simulink model "testEmplanner_cs"  (R2021b)
settings: Solver=ode5  StartTime=0.0  StopTime=60  FixedStep=1/1000  RelTol=1e-3
PreLoadFcn:
  | mbxruntime.callbacks.PreLoadFcn(bdroot);
PostLoadFcn:
  | mbxruntime.callbacks.PostLoadFcn(bdroot);
InitFcn:
  | mbxruntime.callbacks.InitFcn(bdroot);
StartFcn:
  | mbxruntime.callbacks.StartFcn(bdroot);
StopFcn:
  | mbxruntime.callbacks.StopFcn(bdroot);
model workspace (MAT data in the model file):
  mbox_table : object (value not decoded)
  model_closed = 0
  sim_status = 0
values from neighbouring files (symbols this model uses):
  c_factor = 43.75    [emplanner_init.m]
  cf = -175016    [emplanner_init.m]
  cr = -130634    [emplanner_init.m]
  global_path_x = [-1.1448 -0.145417744933 0.852705365581 1.84955224935 2.84511712279 3.83939835808 4.83239585569 5.82411007764 6.81454169183 7.80369144113 8.79156009523 9.77814843293 ... (3001 elements, 3001x1)]    [global_path.mat]
  global_path_y = [14.6488 14.6488 14.6488 14.6488 14.6488 14.6488 14.6488 14.6488 14.6488 14.6488 14.6488 14.6488 ... (3001 elements, 3001x1)]    [global_path.mat]
  KD_PID_distance = 0.0    (= 0)    [emplanner_init.m]
  KD_PID_speed = 0    [emplanner_init.m]
  KI_PID_distance = 0.0    (= 0)    [emplanner_init.m]
  KI_PID_speed = 0    [emplanner_init.m]
  KP_PID_distance = 0.5    [emplanner_init.m]
  KP_PID_speed = 1.8    [emplanner_init.m]
  la = 1.265    [emplanner_init.m]
  lb = 2.947-1.265    (= 1.682)    [emplanner_init.m]
  LQR_K1 = k(:,1)'    [emplanner_init.m]
  LQR_K2 = k(:,2)'    [emplanner_init.m]
  LQR_K3 = k(:,3)'    [emplanner_init.m]
  LQR_K4 = k(:,4)'    [emplanner_init.m]
  m = 2020    [emplanner_init.m]
  rack_displacement = [-39.14 , -37.2 , -35.29 , -33.43 , -31.6 , -29.81 , -28.06 , -26.34 , -24.66 ,      -23.01 , -21.38 , -19.79 , -18.23 , -16.69 , -15.18 , -13.7 , -12.23 , -10.8 , -9.38 , -7.98 ,     -6.61 , -5.25 , -3.91 , -2.59 , -1.29 , 0 , 1.27 , 2.54 , 3.78 , 5.02 , 6.24 , 7.46 , 8.66 ,      9.86 , 11.05 , 12.24 , 13.41 , 14.59 , 15.76 , 16.92 , 18.09 , 19.25 , 20.42 , 21.59 , 22.76 ,      23.93 , 25.11 , 26 ...(+26 chars)    [emplanner_init.m]
  right_wheel_ground = [-70 ,-67.2 , -64.4 , -61.6 , -58.8 , -56 , -53.2 , -50.4 , -47.6 , -44.8 , -42 ,      -39.2 , -36.4 , -33.6 , -30.8 , -28 , -25.2 , -22.4 , -19.6 , -16.8 , -14 , -11.2 , -8.4 , -5.6 ,      -2.8 , 0 , 2.8 , 5.6 , 8.4 , 11.2 , 14 , 16.8 , 19.6 , 22.4 , 25.2 , 28 , 30.8 , 33.6 , 36.4 ,      39.2 , 42 , 44.8 , 47.6 , 50.4 , 53.2 , 56 , 58.8 , 61.6 , 64.4 , 67.2 , 70 ]    [emplanner_init.m]
  vx_break_point = zeros(1,5000)    [emplanner_init.m]
undefined symbols (not defined in the file or in its folder): aubr, DiscIntNeverNeededParam, tablebr, vubr, warningInitialVelocity, x0
libraries: simulink x19, PreScanSimulinkLibrary x17, simulink_extras x6, Solver_SF x1
(part 10 of 14)

== matlab function testEmplanner_cs/Audi_A8_Sedan_1/decision&planning module/EM Planner/decesion task/path decision with dynamic planning(dp) ==
  data: obs_s_set input; dp_path_s output; obs_l_set input; plan_start_s input; plan_start_l input; plan_start_dl input; plan_start_dll input; w_cost_collision input; w_cost_smooth_dl input; w_cost_smooth_ddl input; w_cost_smooth_dddl input; w_cost_ref input; row input; col input; sample_s input; sample_l input; dp_path_l output
function [dp_path_s,dp_path_l] = fcn(obs_s_set,obs_l_set,plan_start_s,plan_start_l,plan_start_dl,...
    plan_start_dll,w_cost_collision,w_cost_smooth_dl,w_cost_smooth_ddl,w_cost_smooth_dddl,w_cost_ref,row,col,sample_s,sample_l)
%该函数为路径决策算法动态规划的主函数
% 输入：obs s l set 筛选后的障碍物sl信息
%       plan_start s l dl ddl 规划起点信息
%       w_cost_obs,w_cost_smooth_dl,w_cost_smooth_ddl,w_cost_smooth_dddl,w_cost_ref动态规划代价权重
%       row col 动态规划采样点的行数和列数(row必须是奇数，col必须是6)
%       sample_s,sample_l 采样的s l 长度
% 输出：dp_path_l,dp_path_s 动态规划的路径sl,此路径不包含规划起点  

%动态规划最优的数据结构是结构体矩阵，但是simulink不支持结构体矩阵，所以动态规划算法写的相对难以理解

%声明二维矩阵变量node_cost，node_cost(i,j)表示从起点出发，到行i列j节点的最小代价为node_cost(i,j)
node_cost = ones(row,col)*inf;%初始化为无穷大

%声明二维矩阵变量pre_node_index pre_node_index(i,j)表示从起点到行i列j的节点的最优路径中前一个节点的行号为
%pre_node_index(i,j)
%例：比如一条最优路径为 起点 -> node(1,1) -> node(2,2) -> node(3,3)
%则pre_node_index(3,3) = 2 (最优路径的前一个节点是node(2,2) 取它的行号）
%  pre_node_index(2,2) = 1 (最优路径的前一个节点是node(1,1) 取它的行号）
%  pre_node_index(1,1) = 0 (起点的行号默认是0)

% 其实pre_node_index就是当找到最小代价的路径后从终点到起点反向选择出最优路径的
%如果用结构体矩阵完全没有必要弄得这么麻烦，但是simulink不支持
pre_node_index = zeros(row,col);%初始化，所有节点的上个最优节点的行号都是0，也就是起点

%先计算从起点到第一列的cost
for i = 1:row
    node_cost(i,1) = CalcStartCost(plan_start_s,plan_start_l,plan_start_dl,...
    plan_start_dll,i,sample_s,sample_l,w_cost_collision,w_cost_smooth_dl,...
    w_cost_smooth_ddl,w_cost_smooth_dddl,w_cost_ref,obs_s_set,obs_l_set,row);
end
% 动态规划主函数，从第二列开始
for j = 2:col
    for i = 1:row
        %计算当前node(i,j)的s l
        cur_node_s = plan_start_s + j * sample_s;
        cur_node_l = ((row + 1)/2 - i) * sample_l;
        %遍历前一列的节点
        for k = 1:row
            %计算前一列节点的s l
            pre_node_s = plan_start_s + (j - 1) * sample_s;
            pre_node_l = ((row + 1)/2 - k) * sample_l;
            cost_neighbour = CalcNeighbourCost(pre_node_s,pre_node_l,cur_node_s,cur_node_l,w_cost_collision,...
    w_cost_smooth_dl,w_cost_smooth_ddl,w_cost_smooth_dddl,w_cost_ref,obs_s_set,obs_l_set);
            %起点到上一个节点的最小代价为node_cost(k,j-1)
            pre_min_cost = node_cost(k,j-1);
            %起点到node_cost(i,j)的最小代价 为node_cost(k,j-1)
            %再加上node(k,j-1)到node(i,j)的代价 (k = 1,2,3,4...row) 中最小的
            cost_temp = pre_min_cost + cost_neighbour;
            if cost_temp < node_cost(i,j)
                node_cost(i,j) = cost_temp;
                %把最优路径上一列节点的行号记录下来
                pre_node_index(i,j) = k;
            end
        end      
    end
end
%找到node_cost最后一列中，cost最小的，记代价最小的行号为index
index = 0;
min_cost = inf;
for i = 1:row
    if node_cost(i,end) < min_cost
        min_cost = node_cost(i,end);
        index = i;
    end
end
%动态规划最优路径初始化
dp_node_list_row = zeros(col,1);
%从后往前逆推
cur_index = index;
for i = 1:col
    %记录cur_index前面节点的行号
    pre_index = pre_node_index(cur_index,end - i + 1);
    %把cur_index放到dp_node_list_row对应的位置
    dp_node_list_row(col - i + 1) = cur_index;
    %再把pre_index 赋给 cur_index 进行下一步递推
    cur_index = pre_index;
end
% 输出初始化，由于事先不知道横纵向的采样列数，因此需要做缓冲
dp_path_s = ones(15,1)*-1;
dp_path_l = ones(15,1)*-1;
for i = 1:col
    dp_path_s(i) = plan_start_s + i * sample_s;
    dp_path_l(i) = ((row + 1) / 2 - dp_node_list_row(i)) * sample_l;
end








end
function cost = CalcNeighbourCost(pre_node_s,pre_node_l,cur_node_s,cur_node_l,w_cost_collision,...
    w_cost_smooth_dl,w_cost_smooth_ddl,w_cost_smooth_dddl,w_cost_ref,obs_s_set,obs_l_set)
% 该函数将计算相邻两个节点之间的cost
  
    start_l = pre_node_l;
    start_dl = 0;
    start_ddl = 0;
    end_l = cur_node_l;
    end_dl = 0;
    end_ddl = 0;
    start_s = pre_node_s;
    end_s = cur_node_s;
    coeff = CalcQuinticCoeffient(start_l,start_dl,start_ddl,end_l,end_dl,end_ddl,start_s,end_s);
    a0 = coeff(1);
    a1 = coeff(2);
    a2 = coeff(3);
    a3 = coeff(4);
    a4 = coeff(5);
    a5 = coeff(6);
    % 取10个点计算cost
    ds = zeros(10,1);
    l = zeros(10,1);
    dl = zeros(10,1);
    ddl = zeros(10,1);
    dddl = zeros(10,1);
    for i = 1:10
        ds(i) = start_s + (i-1)*(end_s - start_s)/10;
    end
    l = a0 * ones(10,1) + a1 * ds + a2 * ds.^2 + a3 * ds.^3 + a4 * ds.^4 + a5 * ds.^5;
    dl = a1 * ones(10,1) + 2 * a2 * ds + 3 * a3 * ds.^2 + 4 * a4 * ds.^3 + 5 * a5 * ds.^4;
    ddl = 2 * a2 * ones(10,1) + 6 * a3 * ds + 12 * a4 * ds.^2 + 20 * a5 * ds.^3;
    dddl = 6 * ones(10,1) * a3 + 24 * a4 * ds + 60 * a5 * ds.^2;
    cost_smooth = w_cost_smooth_dl * (dl' * dl) + w_cost_smooth_ddl * (ddl' * ddl) + w_cost_smooth_dddl * (dddl' * dddl);
    cost_ref = w_cost_ref * (l' * l);
    cost_collision = 0;
    for i = 1:length(obs_s_set)
        if isnan(obs_s_set(i))
            break;
        end
        dlon = ones(10,1) * obs_s_set(i) - ds;
        dlat = ones(10,1) * obs_l_set(i) - l;
        %这里做了非常简化的质点模型，认为障碍物就是一个点
        square_d = dlon.^2 + dlat.^2;
        cost_collision_once = CalcObsCost(w_cost_collision,square_d);
        cost_collision = cost_collision + cost_collision_once;
    end
    cost = cost_collision + cost_smooth + cost_ref;


end


function cost = CalcStartCost(begin_s,begin_l,begin_dl,begin_ddl,cur_node_row,sample_s,sample_l,w_cost_collision,...
    w_cost_smooth_dl,w_cost_smooth_ddl,w_cost_smooth_dddl,w_cost_ref,obs_s_set,obs_l_set,row)
    %该函数将计算起点到第一层的cost
    start_l = begin_l;
    start_dl = begin_dl;
    start_ddl = begin_ddl;
    %  . . .
    %  . . . row = 3 中间的行号 = (row + 1) /2 = 2
    %  . . .
    end_l = ((row + 1)/2 - cur_node_row)*sample_l;
    end_dl = 0;
    end_ddl = 0;
    start_s = begin_s;
    end_s = begin_s + sample_s;
    coeff = CalcQuinticCoeffient(start_l,start_dl,start_ddl,end_l,end_dl,end_ddl,start_s,end_s);
    a0 = coeff(1);
    a1 = coeff(2);
    a2 = coeff(3);
    a3 = coeff(4);
    a4 = coeff(5);
    a5 = coeff(6);
    % 取10个点计算cost
    ds = zeros(10,1);
    l = zeros(10,1);
    dl = zeros(10,1);
    ddl = zeros(10,1);
    dddl = zeros(10,1);
    for i = 1:10
        ds(i) = start_s + (i-1)*sample_s/10;
    end
    l = a0 * ones(10,1) + a1 * ds + a2 * ds.^2 + a3 * ds.^3 + a4 * ds.^4 + a5 * ds.^5;
    dl = a1 * ones(10,1) + 2 * a2 * ds + 3 * a3 * ds.^2 + 4 * a4 * ds.^3 + 5 * a5 * ds.^4;
    ddl = 2 * a2 * ones(10,1) + 6 * a3 * ds + 12 * a4 * ds.^2 + 20 * a5 * ds.^3;
    dddl = 6 * ones(10,1) * a3 + 24 * a4 * ds + 60 * a5 * ds.^2;
    cost_smooth = w_cost_smooth_dl * (dl' * dl) + w_cost_smooth_ddl * (ddl' * ddl) + w_cost_smooth_dddl * (dddl' * dddl);
    cost_ref = w_cost_ref * (l' * l);
    cost_collision = 0;
    for i = 1:length(obs_s_set)
        if isnan(obs_s_set(i))
            break;
        end
        dlon = ones(10,1) * obs_s_set(i) - ds;
        dlat = ones(10,1) * obs_l_set(i) - l;
        %这里做了非常简化的质点模型，认为障碍物就是一个点
        square_d = dlon.^2 + dlat.^2;
        cost_collision_once = CalcObsCost(w_cost_collision,square_d);
        cost_collision = cost_collision + cost_collision_once;
    end
    cost = cost_collision + cost_smooth + cost_ref;
        
end

function obs_cost = CalcObsCost(w_cost_collision,square_d)
%该函数将计算障碍物的距离代价
% 暂定超过4米的cost为0 在4到3米的cost为1000/squard_d,在小于3米的cost为w_cost_collision
  cost = 0;
  for i = 1:length(square_d)
      if (square_d(i) < 16 && square_d(i) > 9) 
          cost = cost + 1000/square_d(i);
      elseif (square_d(i) < 9)
          cost = cost + w_cost_collision;
      end
  end
  obs_cost = cost;

end

function coeff = CalcQuinticCoeffient(start_l,start_dl,start_ddl,end_l,end_dl,end_ddl,start_s,end_s)
    % l = a0 + a1*s + a2*s^2 + a3*s^3 + a4*s^4 + a5*s^5
    % l' = a1 + 2 * a2 * s + 3 * a3 * s^2 + 4 * a4 * s^3 + 5 * a5 * s^4
    % l'' = 2 * a2 + 6 * a3 * s + 12 * a4 * s^2 + 20 * a5 * s^3
    start_s2 = start_s * start_s;
    start_s3 = start_s2 * start_s;
    start_s4 = start_s3 * start_s;
    start_s5 = start_s4 * start_s;
    end_s2 = end_s * end_s;
    end_s3 = end_s2 * end_s;
    end_s4 = end_s3 * end_s;
    end_s5 = end_s4 * end_s;
    A = [1,start_s, start_s2,     start_s3,     start_s4,      start_s5;
         0 1,       2 * start_s,  3 * start_s2, 4 * start_s3,  5 * start_s4;
         0 0,       2,            6 * start_s,  12 * start_s2, 20 * start_s3;
         1,end_s, end_s2,     end_s3,     end_s4,      end_s5;
         0,1,     2 * end_s,  3 * end_s2, 4 * end_s3,  5 * end_s4;
         0,0,     2,          6 * end_s,  12 * end_s2, 20 * end_s3;];
    B = [start_l;
         start_dl;
         start_ddl;
         end_l;
         end_dl;
         end_ddl;];
     coeff = A \ B;
    
end

== matlab function testEmplanner_cs/Audi_A8_Sedan_1/decision&planning module/referenceline provider/MATLAB Function ==
  data: x_set input; match_point_index_set output; y_set input; frenet_path_x input; frenet_path_y input; frenet_path_heading input; frenet_path_kappa input; proj_x_set output; proj_y_set output; proj_heading_set output; proj_kappa_set output
function [match_point_index_set,proj_x_set,proj_y_set,proj_heading_set,proj_kappa_set] = ...
	fcn(x_set,y_set,frenet_path_x,frenet_path_y,frenet_path_heading,frenet_path_kappa)
	
%该函数将批量计算x_set,y_set中(x,y) 在frenet坐标系下的投影信息
%输入： x_set，y_set 待投影的点的集合
	%x_set,y_set,frenet_path_x,frenet_path_y,frenet_path_heading,frenet_path_kappa
	%曲线在直角坐标系下的x,y,heading,kappa
%输出：math_point_index_set 匹配点在frenet_path下的编号的集合（即从全局路径的第一个点开始数，第几个点是匹配点）

%由于事先不知道x_set中有多少个点需要投影，因此事先声明一个最大数量的点作为缓冲

n = 128;
%并且不知道投影点的数量，所以也不知道输出的数量，因此输出也要做缓冲，用nan表示不存在的点
%初始化输出最多为128个点。
%输出初始化
match_point_index_set = ones(n,1) * nan;
proj_x_set = ones(n,1) * nan;
proj_y_set = ones(n,1) * nan;
proj_heading_set = ones(n,1) * nan;
proj_kappa_set = ones(n,1) * nan;

%找匹配点，需要利用上一个周期的结果作为下一个周期遍历的起点，因此需要声明两个全局变量
persistent is_first_run;
persistent pre_match_point_index_set;%bug :pre_match_point_index(i) 未必代表的是第i个障碍物的match_point_index
persistent pre_frenet_path_x;
persistent pre_frenet_path_y;
persistent pre_frenet_path_heading;
persistent pre_frenet_path_kappa;
persistent pre_x_set;
persistent pre_y_set;
%算法主函数入口

if isempty(is_first_run)
	% 该if分支表示函数首次运行
	is_first_run = 0; %赋值
	pre_frenet_path_x = frenet_path_x;
	pre_frenet_path_y = frenet_path_y;
	pre_frenet_path_heading = frenet_path_heading;
	pre_frenet_path_kappa = frenet_path_kappa;
	%记录首次运行计算的匹配点的结果供下个周期运行，先初始化
	pre_match_point_index_set = ones(n,1) * nan;
	
	%对x_set,y_set的点做遍历，找到他们的匹配点
	for i = 1 : length(x_set)
        if isnan(x_set(i))
            break;
        end
	%首次运行时，没有任何提示，只能从frenet_path的第一个点开始找
	start_search_index = 1;
	%声明increa_count,用于表示在遍历时distance连续增大的次数
	increase_count = 0;
	%开始遍历
	min_distance = inf;
	for j = start_search_index : length(frenet_path_x)
		distance = (x_set(i) - frenet_path_x(j))^2 + (y_set(i) - frenet_path_y(j))^2;
		%处理最小值
		if distance < min_distance
			min_distance = distance;
			match_point_index_set(i) = j; %math_point_index_set存放匹配点的序号
			increase_count = 0;
		else
			increase_count = increase_count + 1;
		end
		% 如果连续distanc增加50次,就不要再遍历了，节省时间
		if increase_count > 50 
			break;
		end	
	end
	%如何通过匹配点计算投影点，参考《自动驾驾驶控制算法第七讲》
	%或者《自动驾驶决策规划算法》第一章第三节
		
	%取出匹配点的编号
	match_point_index = match_point_index_set(i);
		
	%取出匹配点信息
	match_point_x = frenet_path_x(match_point_index);
	match_point_y = frenet_path_y(match_point_index);
	match_point_heading = frenet_path_heading(match_point_index);
	match_point_kappa = frenet_path_kappa(match_point_index);
		
	% 计算匹配点的位置向量和方向向量
	vector_match_point = [match_point_x;match_point_y];%位置向量
	vector_match_point_direction = [cos(match_point_heading);sin(match_point_heading)];%方向向量，全局坐标系下（大地坐标系）
		
	%声明待投影点的位矢
	vector_r = [x_set(i);y_set(i)];
		
	%通过匹配点计算投影点
	vector_d = vector_r - vector_match_point;
	ds = vector_d' * vector_match_point_direction;
	vector_proj_point = vector_match_point + ds * vector_match_point_direction;
	proj_heading = match_point_heading + match_point_kappa * ds;
	proj_kappa = match_point_kappa;
		
	%计算结果输出 
	proj_x_set(i) = vector_proj_point(1);
	proj_y_set(i) = vector_proj_point(2);
	proj_heading_set(i) = proj_heading;
	proj_kappa_set(i) = proj_kappa;
   end
	
	%匹配点的计算结果保存，供下一个周期使用
	pre_match_point_index_set = match_point_index_set;
	pre_x_set = x_set;
	pre_y_set = y_set;
else
	% 此分支不是首次运行
	
	%对每个x_set上的点做处理
	for i = 1 : length(x_set)
		%不是首次运行，对于点x_set(i),y_set(i)来说，
		%start_search_index = pre_match_point_index_set(i)
		start_search_index = pre_match_point_index_set(i);%上个周期匹配点的编号作为本周期搜索的起点
		%判断帧与帧之间的障碍物是否为同一个
		square_dis = (x_set(i) - pre_x_set(i))^2 + (y_set(i) - pre_y_set(i))^2;
		if square_dis > 36	 
			% 帧与帧之间的物体位置距离过大，认为是两个障碍物
			start_search_index = nan;
		end
        %
        % 对于障碍物的检测而言，当感知第一次检测到障碍物时，算法并不是首次运行，此时
        % pre_match_point_set的值是nan，如果还用上一个时刻的结果作为本周期搜索的起点
        % 必然会出问题，所以要修改
        % 声明 increase_count_limit
        increase_count_limit = 5;
        if isnan(start_search_index)
	        % 没有上个周期的结果，那么就不能只检查5次
	        increase_count_limit = 50;
	        % 搜索的起点也要设为 1
	        start_search_index = 1;
        end
		%声明increa_count,用于表示在遍历时distance连续增大的次数
		increase_count = 0;
		%开始遍历
		
		%这里多了一个步骤，判断遍历的方向
		%计算上个周期匹配点的位失
		vector_pre_match_point = [pre_frenet_path_x(start_search_index); pre_frenet_path_y(start_search_index)];
		vector_pre_match_point_direction = ...
			[cos(pre_frenet_path_heading(start_search_index));sin(pre_frenet_path_heading(start_search_index))];
		
		% 判断遍历的方向
		flag = ([x_set(i);y_set(i)] - vector_pre_match_point)' * vector_pre_match_point_direction;
		
		min_distance = inf;
		
		if flag > 0.001 
			for j = start_search_index : length(frenet_path_x)
				distance = (x_set(i) - frenet_path_x(j))^2 + (y_set(i) - frenet_path_y(j))^2;
				%处理最小值
				if distance < min_distance
					min_distance = distance;
					match_point_index_set(i) = j; %math_point_index_set存放匹配点的序号
					increase_count = 0;
				else
					increase_count = increase_count + 1;
				end
				% 如果连续distanc增加increase_count_limit次,就不要再遍历了，节省时间
				if increase_count > increase_count_limit
					break;
				end
			end
		elseif flag < -0.001
			for j = start_search_index :-1: 1
				distance = (x_set(i) - frenet_path_x(j))^2 + (y_set(i) - frenet_path_y(j))^2;
				%处理最小值
				if distance < min_distance
					min_distance = distance;
					match_point_index_set(i) = j; %math_point_index_set存放匹配点的序号
					increase_count = 0;
				else
					increase_count = increase_count + 1;
				end
				% 如果连续distanc增加50次,就不要再遍历了，节省时间
				if increase_count > increase_count_limit 
					break;
				end
			end
		else
			match_point_index_set(i) = start_search_index;
		end
			
		%如何通过匹配点计算投影点，参考《自动驾驾驶控制算法第七讲》
		%或者《自动驾驶决策规划算法》第一章第三节
		
		%取出匹配点的编号
		match_point_index = match_point_index_set(i);
		
		%取出匹配点信息
		match_point_x = frenet_path_x(match_point_index);
		match_point_y = frenet_path_y(match_point_index);
		match_point_heading = frenet_path_heading(match_point_index);
		match_point_kappa = frenet_path_kappa(match_point_index);
		
		% 计算匹配点的位置向量和方向向量
		vector_match_point = [match_point_x;match_point_y];%位置向量
		vector_match_point_direction = [cos(match_point_heading);sin(match_point_heading)];%方向向量
		
		%声明待投影点的位矢
		vector_r = [x_set(i);y_set(i)];
		
		%通过匹配点计算投影点
		vector_d = vector_r - vector_match_point;
		ds = vector_d' * vector_match_point_direction;
		vector_proj_point = vector_match_point + ds * vector_match_point_direction;
		proj_heading = match_point_heading + match_point_kappa * ds;
		proj_kappa = match_point_kappa;
		
		%计算结果输出 
		proj_x_set(i) = vector_proj_point(1);
		proj_y_set(i) = vector_proj_point(2);
		proj_heading_set(i) = proj_heading;
		proj_kappa_set(i) = proj_kappa;
	end
	
	%匹配点的计算结果保存，供下一个周期使用
	pre_match_point_index_set = match_point_index_set;
	pre_frenet_path_x = frenet_path_x;
	pre_frenet_path_y = frenet_path_y;
	pre_frenet_path_heading = frenet_path_heading;
	pre_frenet_path_kappa = frenet_path_kappa;
	pre_x_set = x_set;
	pre_y_set = y_set;
end

== matlab function testEmplanner_cs/Audi_A8_Sedan_1/decision&planning module/EM Planner/decesion task/increase DP path nodes ==
  data: dp_path_s_init input; dp_path_s_final output; dp_path_l_init input; plan_start_s input; plan_start_l input; plan_start_dl input; plan_start_ddl input; dp_path_l_final output; dp_path_dl_final output; dp_path_ddl_final output
function [dp_path_s_final,dp_path_l_final,dp_path_dl_final,dp_path_ddl_final] = ... 
	fcn(dp_path_s_init,dp_path_l_init,plan_start_s,plan_start_l,plan_start_dl,plan_start_ddl)
% 该函数将增密dp_path_s,dp_path_l
% 由于事先不知道动态规划采样的行和列，也就不知道动态规划计算的曲线有多长，因此需要做缓冲
% 每1“米” 采样一个点，一共60个
ds = 1;
% 输出初始化
dp_path_s_final = ones(60,1) * nan;
dp_path_l_final = ones(60,1) * nan;
dp_path_dl_final = ones(60,1) * nan;
dp_path_ddl_final = ones(60,1) * nan;

% 设置五次多项式的起点
start_s = plan_start_s;
start_l = plan_start_l;
start_dl = plan_start_dl;
start_ddl = plan_start_ddl;

s_cur = [];
l_temp = [];
dl_temp = [];
ddl_temp = [];

for i = 1 : length(dp_path_s_init)
	if isnan(dp_path_s_init(i)) 
		break;
	end
	for j = 1 : 1000
		% 采样s
		s_node = start_s + ds * (j - 1);
		if s_node < dp_path_s_init(i)
			s_cur = [s_cur,s_node];% 矩阵动态扩容
		else
			break;
		end

	end
	end_s = dp_path_s_init(i);
	end_l = dp_path_l_init(i);
	end_dl = 0;
	end_ddl = 0;
	coeff = CalcQuinticCoeffient(start_l,start_dl,start_ddl,end_l,end_dl,end_ddl,start_s,end_s);
	a0 = coeff(1);
	a1 = coeff(2);
	a2 = coeff(3);
	a3 = coeff(4);
	a4 = coeff(5);
	a5 = coeff(6);
	l = a0 * ones(1,length(s_cur)) + a1 * s_cur + a2 * s_cur.^2 + a3 * s_cur.^3 +...
		a4 * s_cur.^4 + a5 * s_cur.^5 ;
	dl = a1 * ones(1,length(s_cur)) + 2 * a2 * s_cur + 3 * a3 * s_cur.^2 + ...
		4 * a4 * s_cur.^3 + 5 * a5 * s_cur.^4;
	ddl = 2 * a2 * ones(1,length(s_cur)) + 6 * a3 * s_cur + ...
		12 * a4 * s_cur.^2 + 20 * a5 * s_cur.^3;
	% 把 l dl ddl 的结果保存
	l_temp = [l_temp,l];
	dl_temp = [dl_temp,dl];
	ddl_temp = [ddl_temp,ddl];
	% end的值 赋值给start做下一步循环使用
	start_s = end_s;
	start_l = end_l;
	start_dl = end_dl;
	start_ddl = end_ddl;
	s_cur = [];% 清空临时数组
end

	for k = 1 : length(l_temp)
		if k == 61 
			break;
		end

		dp_path_s_final(k) = plan_start_s + ds * (k - 1);
		dp_path_l_final(k) = l_temp(k);
		dp_path_dl_final(k) = dl_temp(k);
		dp_path_ddl_final(k) = ddl_temp(k);

	end

end


function coeff = CalcQuinticCoeffient(start_l,start_dl,start_ddl,end_l,end_dl,end_ddl,start_s,end_s)
	% l = a0 + a1 * s + a2 * s^2 + a3 * s^3 + a4 * s^4 + a5 * s^5;
	% l' = a1 + 2 * a2 * s + 3 * a3 * s^2 + 4 * a4 * s^3 + 5 * a5 * s^4;
	% l'' = 2 * a2 + 6 * a3 * s + 12 * a4 * s^2 + 20 * a5 * s^3;
	start_s2 = start_s * start_s;
	start_s3 = start_s2 * start_s;
	start_s4 = start_s3 * start_s;
	start_s5 = start_s4 * start_s;

	end_s2 = end_s * end_s;
	end_s3 = end_s2 * end_s;
	end_s4 = end_s3 * end_s;
	end_s5 = end_s4 * end_s;
	% 构造A B矩阵，然后求方程的系数即可

	A = [ 1, start_s, start_s2,  start_s3,   start_s4,   start_s5;
		  0 , 1     , 2*start_s, 3*start_s2, 4*start_s3,  5*start_s4;
		  0 , 0     , 2        , 6*start_s,  12*start_s2, 20*start_s3;
		  1, end_s, end_s2,  end_s3,   end_s4,   end_s5;
		  0 , 1     , 2*end_s, 3*end_s2, 4*end_s3,  5*end_s4;
		  0 , 0     , 2       , 6*end_s,  12*end_s2, 20*end_s3;
		];
	B = [ start_l;
		  start_dl;
		  start_ddl;
		  end_l;
		  end_dl;
		  end_ddl;
		];
	coeff = A \ B;
end

== matlab function testEmplanner_cs/Audi_A8_Sedan_1/decision&planning module/EM Planner/MATLAB Function3 ==
  data: dp_speed_s input; dp_speed_t input; qp_speed_s input; qp_speed_t input; obs_s_in_set input; obs_s_out_set input; obs_t_in_set input; obs_t_out_set input
function  fcn(dp_speed_s,dp_speed_t,qp_speed_s,qp_speed_t,obs_s_in_set,obs_s_out_set,obs_t_in_set,obs_t_out_set)
coder.extrinsic("plot");
cla;
n = length(dp_speed_s);
m = length(obs_s_in_set);
s = length(qp_speed_s);
for i = 1:length(dp_speed_s)
    if isnan(dp_speed_s(i))
        n = i -1;
        break;
    end
end
for i = 1:length(qp_speed_s)
    if isnan(qp_speed_s(i))
        s = i -1;
        break;
    end
end

plot(dp_speed_t(1:n),dp_speed_s(1:n),'r')
plot(qp_speed_t(1:s),qp_speed_s(1:s),'b')
hold on
axis([-1 10 -10 50]);
for i = 1:m
    if isnan(obs_s_in_set(i))
        continue;
    end
    point_t = [obs_t_in_set(i),obs_t_out_set(i)];
    point_s = [obs_s_in_set(i),obs_s_out_set(i)];
    plot(point_t,point_s)
end

== matlab function testEmplanner_cs/Audi_A8_Sedan_1/decision&planning module/EM Planner/MATLAB Function5 ==
  data: x_set input; match_point_index_set output; y_set input; frenet_path_x input; frenet_path_y input; frenet_path_heading input; frenet_path_kappa input; proj_x_set output; proj_y_set output; proj_heading_set output; proj_kappa_set output
function [match_point_index_set,proj_x_set,proj_y_set,proj_heading_set,proj_kappa_set] = ...
	fcn(x_set,y_set,frenet_path_x,frenet_path_y,frenet_path_heading,frenet_path_kappa)
	
%该函数将批量计算x_set,y_set中(x,y) 在frenet坐标系下的投影信息
%输入： x_set，y_set 待投影的点的集合
	%x_set,y_set,frenet_path_x,frenet_path_y,frenet_path_heading,frenet_path_kappa
	%曲线在直角坐标系下的x,y,heading,kappa
%输出：math_point_index_set 匹配点在frenet_path下的编号的集合（即从全局路径的第一个点开始数，第几个点是匹配点）

%由于事先不知道x_set中有多少个点需要投影，因此事先声明一个最大数量的点作为缓冲

n = 128;
%并且不知道投影点的数量，所以也不知道输出的数量，因此输出也要做缓冲，用nan表示不存在的点
%初始化输出最多为128个点。
%输出初始化
match_point_index_set = ones(n,1) * nan;
proj_x_set = ones(n,1) * nan;
proj_y_set = ones(n,1) * nan;
proj_heading_set = ones(n,1) * nan;
proj_kappa_set = ones(n,1) * nan;

%找匹配点，需要利用上一个周期的结果作为下一个周期遍历的起点，因此需要声明两个全局变量
persistent is_first_run;
persistent pre_match_point_index_set;%bug :pre_match_point_index(i) 未必代表的是第i个障碍物的match_point_index
persistent pre_frenet_path_x;
persistent pre_frenet_path_y;
persistent pre_frenet_path_heading;
persistent pre_frenet_path_kappa;
persistent pre_x_set;
persistent pre_y_set;
%算法主函数入口

if isempty(is_first_run)
	% 该if分支表示函数首次运行
	is_first_run = 0; %赋值
	pre_frenet_path_x = frenet_path_x;
	pre_frenet_path_y = frenet_path_y;
	pre_frenet_path_heading = frenet_path_heading;
	pre_frenet_path_kappa = frenet_path_kappa;
	%记录首次运行计算的匹配点的结果供下个周期运行，先初始化
	pre_match_point_index_set = ones(n,1) * nan;
	
	%对x_set,y_set的点做遍历，找到他们的匹配点
	for i = 1 : length(x_set)
        if isnan(x_set(i))
            break;
        end
	%首次运行时，没有任何提示，只能从frenet_path的第一个点开始找
	start_search_index = 1;
	%声明increa_count,用于表示在遍历时distance连续增大的次数
	increase_count = 0;
	%开始遍历
	min_distance = inf;
	for j = start_search_index : length(frenet_path_x)
		distance = (x_set(i) - frenet_path_x(j))^2 + (y_set(i) - frenet_path_y(j))^2;
		%处理最小值
		if distance < min_distance
			min_distance = distance;
			match_point_index_set(i) = j; %math_point_index_set存放匹配点的序号
			increase_count = 0;
		else
			increase_count = increase_count + 1;
		end
		% 如果连续distanc增加50次,就不要再遍历了，节省时间
		if increase_count > 50 
			break;
		end	
	end
	%如何通过匹配点计算投影点，参考《自动驾驾驶控制算法第七讲》
	%或者《自动驾驶决策规划算法》第一章第三节
		
	%取出匹配点的编号
	match_point_index = match_point_index_set(i);
		
	%取出匹配点信息
	match_point_x = frenet_path_x(match_point_index);
	match_point_y = frenet_path_y(match_point_index);
	match_point_heading = frenet_path_heading(match_point_index);
	match_point_kappa = frenet_path_kappa(match_point_index);
		
	% 计算匹配点的位置向量和方向向量
	vector_match_point = [match_point_x;match_point_y];%位置向量
	vector_match_point_direction = [cos(match_point_heading);sin(match_point_heading)];%方向向量，全局坐标系下（大地坐标系）
		
	%声明待投影点的位矢
	vector_r = [x_set(i);y_set(i)];
		
	%通过匹配点计算投影点
	vector_d = vector_r - vector_match_point;
	ds = vector_d' * vector_match_point_direction;
	vector_proj_point = vector_match_point + ds * vector_match_point_direction;
	proj_heading = match_point_heading + match_point_kappa * ds;
	proj_kappa = match_point_kappa;
		
	%计算结果输出 
	proj_x_set(i) = vector_proj_point(1);
	proj_y_set(i) = vector_proj_point(2);
	proj_heading_set(i) = proj_heading;
	proj_kappa_set(i) = proj_kappa;
   end
	
	%匹配点的计算结果保存，供下一个周期使用
	pre_match_point_index_set = match_point_index_set;
	pre_x_set = x_set;
	pre_y_set = y_set;
else
	% 此分支不是首次运行
	
	%对每个x_set上的点做处理
	for i = 1 : length(x_set)
		%不是首次运行，对于点x_set(i),y_set(i)来说，
		%start_search_index = pre_match_point_index_set(i)
		start_search_index = pre_match_point_index_set(i);%上个周期匹配点的编号作为本周期搜索的起点
		%判断帧与帧之间的障碍物是否为同一个
		square_dis = (x_set(i) - pre_x_set(i))^2 + (y_set(i) - pre_y_set(i))^2;
		if square_dis > 36	 
			% 帧与帧之间的物体位置距离过大，认为是两个障碍物
			start_search_index = nan;
		end
        %
        % 对于障碍物的检测而言，当感知第一次检测到障碍物时，算法并不是首次运行，此时
        % pre_match_point_set的值是nan，如果还用上一个时刻的结果作为本周期搜索的起点
        % 必然会出问题，所以要修改
        % 声明 increase_count_limit
        increase_count_limit = 5;
        if isnan(start_search_index)
	        % 没有上个周期的结果，那么就不能只检查5次
	        increase_count_limit = 50;
	        % 搜索的起点也要设为 1
	        start_search_index = 1;
        end
		%声明increa_count,用于表示在遍历时distance连续增大的次数
		increase_count = 0;
		%开始遍历
		
		%这里多了一个步骤，判断遍历的方向
		%计算上个周期匹配点的位失
		vector_pre_match_point = [pre_frenet_path_x(start_search_index); pre_frenet_path_y(start_search_index)];
		vector_pre_match_point_direction = ...
			[cos(pre_frenet_path_heading(start_search_index));sin(pre_frenet_path_heading(start_search_index))];
		
		% 判断遍历的方向
		flag = ([x_set(i);y_set(i)] - vector_pre_match_point)' * vector_pre_match_point_direction;
		
		min_distance = inf;
		
		if flag > 0.001 
			for j = start_search_index : length(frenet_path_x)
				distance = (x_set(i) - frenet_path_x(j))^2 + (y_set(i) - frenet_path_y(j))^2;
				%处理最小值
				if distance < min_distance
					min_distance = distance;
					match_point_index_set(i) = j; %math_point_index_set存放匹配点的序号
					increase_count = 0;
				else
					increase_count = increase_count + 1;
				end
				% 如果连续distanc增加increase_count_limit次,就不要再遍历了，节省时间
				if increase_count > increase_count_limit
					break;
				end
			end
		elseif flag < -0.001
			for j = start_search_index :-1: 1
				distance = (x_set(i) - frenet_path_x(j))^2 + (y_set(i) - frenet_path_y(j))^2;
				%处理最小值
				if distance < min_distance
					min_distance = distance;
					match_point_index_set(i) = j; %math_point_index_set存放匹配点的序号
					increase_count = 0;
				else
					increase_count = increase_count + 1;
				end
				% 如果连续distanc增加50次,就不要再遍历了，节省时间
				if increase_count > increase_count_limit 
					break;
				end
			end
		else
			match_point_index_set(i) = start_search_index;
		end
			
		%如何通过匹配点计算投影点，参考《自动驾驾驶控制算法第七讲》
		%或者《自动驾驶决策规划算法》第一章第三节
		
		%取出匹配点的编号
		match_point_index = match_point_index_set(i);
		
		%取出匹配点信息
		match_point_x = frenet_path_x(match_point_index);
		match_point_y = frenet_path_y(match_point_index);
		match_point_heading = frenet_path_heading(match_point_index);
		match_point_kappa = frenet_path_kappa(match_point_index);
		
		% 计算匹配点的位置向量和方向向量
		vector_match_point = [match_point_x;match_point_y];%位置向量
		vector_match_point_direction = [cos(match_point_heading);sin(match_point_heading)];%方向向量
		
		%声明待投影点的位矢
		vector_r = [x_set(i);y_set(i)];
		
		%通过匹配点计算投影点
		vector_d = vector_r - vector_match_point;
		ds = vector_d' * vector_match_point_direction;
		vector_proj_point = vector_match_point + ds * vector_match_point_direction;
		proj_heading = match_point_heading + match_point_kappa * ds;
		proj_kappa = match_point_kappa;
		
		%计算结果输出 
		proj_x_set(i) = vector_proj_point(1);
		proj_y_set(i) = vector_proj_point(2);
		proj_heading_set(i) = proj_heading;
		proj_kappa_set(i) = proj_kappa;
	end
	
	%匹配点的计算结果保存，供下一个周期使用
	pre_match_point_index_set = match_point_index_set;
	pre_frenet_path_x = frenet_path_x;
	pre_frenet_path_y = frenet_path_y;
	pre_frenet_path_heading = frenet_path_heading;
	pre_frenet_path_kappa = frenet_path_kappa;
	pre_x_set = x_set;
	pre_y_set = y_set;
end

== matlab function testEmplanner_cs/Audi_A8_Sedan_1/decision&planning module/EM Planner/Frenet2Cartesian ==
  data: s_set input; x_set output; l_set input; dl_set input; ddl_set input; frenet_path_x input; frenet_path_y input; frenet_path_heading input; frenet_path_kappa input; index2s input; y_set output; heading_set output; kappa_set output
function [x_set,y_set,heading_set,kappa_set] = ...
    fcn(s_set,l_set,dl_set,ddl_set,frenet_path_x,frenet_path_y,frenet_path_heading,frenet_path_kappa,index2s)
% 通用算法 frenet转frenet
% 由于不知道有多少个(s,l)要转化成直角坐标，因此做缓冲
% 输出初始化
    x_set = ones(600,1) * nan;
    y_set = ones(600,1) * nan;
    heading_set = ones(600,1) * nan;
    kappa_set = ones(600,1) * nan;
    for i = 1:length(s_set)
        if isnan(s_set(i))
            break;
        end
        % 计算(s,l)在frenet坐标轴上的投影
        [proj_x,proj_y,proj_heading,proj_kappa] = CalcProjPoint(s_set(i),frenet_path_x,frenet_path_y,frenet_path_heading,...
    frenet_path_kappa,index2s);
        nor = [-sin(proj_heading);cos(proj_heading)];
        point = [proj_x;proj_y] + l_set(i) * nor;
        x_set(i) = point(1);
        y_set(i) = point(2);
        heading_set(i) = proj_heading + atan(dl_set(i)/(1 - proj_kappa * l_set(i)));
        % 近似认为 kappa' == 0,frenet转cartesian公式，见第一章第三节评论区的链接
        kappa_set(i) = ((ddl_set(i) + proj_kappa * dl_set(i) * tan(heading_set(i) - proj_heading)) * ...
            (cos(heading_set(i) - proj_heading)^2)/(1 - proj_kappa * l_set(i)) + proj_kappa) * ...
            cos(heading_set(i) - proj_heading)/(1 - proj_kappa * l_set(i));
         
    end

end


function [proj_x,proj_y,proj_heading,proj_kappa] = CalcProjPoint(s,frenet_path_x,frenet_path_y,frenet_path_heading,...
    frenet_path_kappa,index2s)
% 该函数将计算在frenet坐标系下，点(s,l)在frenet坐标轴的投影的直角坐标(proj_x,proj_y,proj_heading,proj_kappa)'
% 先找匹配点的编号
    match_index = 1;
    while index2s(match_index) < s
        match_index = match_index + 1;
    end
    match_point = [frenet_path_x(match_index);frenet_path_y(match_index)];
    match_point_heading = frenet_path_heading(match_index);
    match_point_kappa = frenet_path_kappa(match_index);
    ds = s - index2s(match_index);
    match_tor = [cos(match_point_heading);sin(match_point_heading)];
    proj_point = match_point + ds * match_tor;
    proj_heading = match_point_heading + ds * match_point_kappa;
    proj_kappa = match_point_kappa;
    proj_x = proj_point(1);
    proj_y = proj_point(2);   
end

== matlab function testEmplanner_cs/Audi_A8_Sedan_1/decision&planning module/EM Planner/calc path length and map between point and s ==
  data: trajectory_x input; path_s_end output; trajectory_y input; path_s output
function [path_s_end,path_s] = fcn(trajectory_x,trajectory_y)
% 该函数将计算以trajectory的s 与 x y 的对应关系，可以看作是trajectory index2s
n = length(trajectory_x);
path_s = zeros(n,1);
sum = 0;
for i = 2:length(trajectory_x)
    if isnan(trajectory_x(i))
        break;
    end
    sum = sum + sqrt((trajectory_x(i) - trajectory_x(i-1))^2 + (trajectory_y(i) - trajectory_y(i-1))^2);
    path_s(i) = sum;
end
% 计算出trajectory的长度
if i == n
    path_s_end = path_s(end);
else
    % 因为循环的退出条件为isnan(trajectory_x(i)) 所以 i 所对应的数为 nan 
    path_s_end = path_s(i - 1);
end

== matlab function testEmplanner_cs/Audi_A8_Sedan_1/decision&planning module/EM Planner/calc plan start info gcs ==
  data: pre_trajectory_x input; plan_start_x output; pre_trajectory_y input; pre_trajectory_heading input; pre_trajectory_kappa input; pre_trajectory_velocity input; pre_trajectory_accel input; pre_trajectory_time input; current_time input; host_x input; host_y input; host_heading_xy input; host_vx input; host_vy input; host_ax input; host_ay input; plan_start_y output; plan_start_heading output; plan_start_kappa output; plan_start_vx output; plan_start_vy output; plan_start_ax output; plan_start_ay output; plan_start_time output; stitch_x output; stitch_y output; stitch_heading output; stitch_kappa output; stitch_speed output; stitch_accel output; stitch_time output
function [plan_start_x,plan_start_y,plan_start_heading,plan_start_kappa,plan_start_vx,plan_start_vy,plan_start_ax,...
	plan_start_ay,plan_start_time,stitch_x,stitch_y,stitch_heading,stitch_kappa,stitch_speed,stitch_accel,stitch_time] ...
	= fcn(pre_trajectory_x,pre_trajectory_y,pre_trajectory_heading,pre_trajectory_kappa,pre_trajectory_velocity,...
	pre_trajectory_accel,pre_trajectory_time,current_time,host_x,host_y,host_heading_xy,host_vx,host_vy,host_ax,host_ay)

% 该函数将计算规划的起点以及拼接轨迹的信息
% 输入: 上一个周期的规划结果信息 pre_trajectory x,y,heading,kappa,velocity,accel,time
%       本周期的绝对时间current_time
%       定位信息host_x,y,heading,kappa,vx,vy,ax,ay
% 输出：规划起点信息 plan_start x,y,heading,kappa,vx,vy,ax,ay(vx,vy,ax,ay)是世界坐标系
% 		待规划的轨迹信息，一般在上一个周期的轨迹中的current_time + 100ms,往前取20个点。
%       当规划完成后，本周期的规划结果和stitch_trajectory一起拼好发给控制。


% 输出初始化
stitch_x = zeros(20,1);
stitch_y = zeros(20,1);
stitch_heading = zeros(20,1);
stitch_kappa = zeros(20,1);
stitch_speed = zeros(20,1);
stitch_accel = zeros(20,1);
% 时间为负 代表没有对应拼接的轨迹
stitch_time = ones(20,1) * -1;


% 申明全局变量
persistent is_first_run;
if isempty(is_first_run)
	%代表代码首次运行
	is_first_run = 0;
	%按照百度的工程师的说法，应该用车辆动力学递推，但是首次运行的车辆速度都是0，所以没必要递推了。
	plan_start_x = host_x;
	plan_start_y = host_y;
	plan_start_heading = host_heading_xy;
	plan_start_kappa = 0;
	plan_start_vx = 0;
	plan_start_vy = 0;
	plan_start_ax = 0;
	plan_start_ay = 0;
	% 规划的起点的时间是当前的时间 + 100ms
	plan_start_time = current_time + 0.1;
	
else

	% 该函数不是首次运行
	x_cur = host_x;
	y_cur = host_y;
	heading_cur = host_heading_xy;
	kappa_cur = 0;
	% vx vy ax ay 要转换成世界坐标系
	vx_cur = host_vx * cos(heading_cur) - host_vy * sin(heading_cur);
	vy_cur = host_vx * sin(heading_cur) + host_vy * cos(heading_cur);
	ax_cur = host_ax * cos(heading_cur) - host_ay * sin(heading_cur);
	ay_cur = host_ax * sin(heading_cur) + host_ay * cos(heading_cur);
	% 规划周期 
	dt = 0.1;
	% 由于不是首次运行了，有了上一时刻的轨迹，找到上一周期的轨迹规划的本周期车辆应该在的位置
	for i = 1: length(pre_trajectory_time) - 1
		if(pre_trajectory_time(i) <= current_time && pre_trajectory_time(i+1) > current_time)
			break;
		end
	end
	% 上一周期规划的本周期车应该在的位置
	pre_x_desire = pre_trajectory_x(i);
	pre_y_desire = pre_trajectory_y(i);
	pre_heading_desire = pre_trajectory_heading(i);
	
	%计算横纵向误差
	
	%切向量
	tor = [cos(pre_heading_desire);sin(pre_heading_desire)];
	% 法向量
	nor = [-sin(pre_heading_desire);cos(pre_heading_desire)];
	% 误差向量 
	d_err = [host_x;host_y] - [pre_x_desire;pre_y_desire];
	% 纵向误差
	lon_err = abs(d_err' * tor);
	% 横向误差
	lat_err = abs(d_err' * nor);
	% 纵向误差大于2.5. 横向误差大于0.5 认为控制没有跟上 通过运动学公式递推
	if (lon_err > 2.5) || (lat_err > 0.5)
		%此分支处理控制没有跟上的情况
		plan_start_x = x_cur + vx_cur * dt + 0.5 * ax_cur * dt * dt; 
		plan_start_y = y_cur + vx_cur * dt + 0.5 * ay_cur * dt * dt;
		plan_start_vx = vx_cur + ax_cur * dt;
		plan_start_vy = vy_cur + ay_cur * dt;
		plan_start_heading = atan2(plan_start_vy,plan_start_vx); %%%%%%
		plan_start_ax = ax_cur;
		plan_start_ay = ay_cur;
		plan_start_kappa = kappa_cur;
		plan_start_time = current_time + 0.1;
		return;
	else
		%此分支表示控制能跟上规划，开始拼接
		for j = 1 : length(pre_trajectory_time) - 1 
			if (pre_trajectory_time(j) <= current_time + 0.1 )&& (pre_trajectory_time(j+1) > current_time + 0.1)
				break;
			end
		end
		% 注：此算法要是能运行需要 trajectory 的点有很高的密度
		plan_start_x = pre_trajectory_x(j);
		plan_start_y = pre_trajectory_y(j);
		plan_start_heading  = pre_trajectory_heading(j);
		plan_start_kappa = pre_trajectory_kappa(j);
		% 这里的pre_trajectory 的速度加速度是指轨迹的切向速度，切向加速度
		plan_start_vx = pre_trajectory_velocity(j) * cos(plan_start_heading);
		plan_start_vy = pre_trajectory_velocity(j) * sin(plan_start_heading);
	
		%% pre_trajectiory的加速度是切向加速度，要想计算ax ay，还要计算法向加速度
		%计算轨迹在current_time + 100ms 这个点的切向量 法向量
		tor = [cos(plan_start_heading); sin(plan_start_heading)];
		nor = [-sin(plan_start_heading); cos(plan_start_heading)];
		a_tor = pre_trajectory_accel(j) * tor;
		a_nor = pre_trajectory_velocity(j)^2 * plan_start_kappa * nor;
		plan_start_ax = a_tor(1) + a_nor(1);
		plan_start_ay = a_tor(2) + a_nor(2);
		plan_start_time = pre_trajectory_time(j);
		
		% 计算拼接轨迹 
		% j 表示current_time + 0.1 的时间点在 pre_trajectory_time的编号
		% 拼接是往从j开始，往前拼接20个点，也就是pre_trajectory(j-1),j-2,j-3,...,j-19
		% 分两种情况，如果j小于20,意味着前面的轨迹点不够20个
		% 如果j >= 20 意味着前面的点多余20个
		% 还有一个细节需要考虑，pre_trajectory x(j) y(j) ... 是规划的起点，那么轨迹拼接时，需不需要在
		% stitch_trajectory 中把pre_trajectory x(j) y(j) ... 包含进去
		% 答案是否定的，不应该包进去，因为规划的起点会在规划模块计算完成后的结果中包含，如果在拼接的时候还要包含，
		% 那就等于规划的起点包含了两次
		% 除非本周期计算的轨迹不包含规划的起点，那么stitch_trajectory可以包含规划的起点
		% 如果本周期计算的轨迹包含规划的起点，那么stitch_trajectory就不包含规划的起点
		% 我们选择规划包含起点，拼接不包含起点的做法
		
		% 把起点去掉
		
		j = j-1;
		if j >= 20 
			stitch_x = pre_trajectory_x(j - 19:j);
			stitch_y = pre_trajectory_y(j - 19:j);
			stitch_heading = pre_trajectory_heading(j - 19:j);
			stitch_kappa = pre_trajectory_kappa(j - 19:j);
			stitch_speed = pre_trajectory_velocity(j - 19:j);
			stitch_accel = pre_trajectory_accel(j - 19:j);
			stitch_time = pre_trajectory_time(j - 19:j);
		else
			stitch_x(20 -j + 1:20) = pre_trajectory_x(1:j);
			stitch_y(20 -j + 1:20) = pre_trajectory_y(1:j);
			stitch_heading(20 -j + 1:20) = pre_trajectory_heading(1:j);
			stitch_kappa(20 -j + 1:20) = pre_trajectory_kappa(1:j);
			stitch_speed(20 -j + 1:20) = pre_trajectory_velocity(1:j);
			stitch_accel(20 -j + 1:20) = pre_trajectory_accel(1:j);
			stitch_time(20 -j + 1:20) = pre_trajectory_time(1:j);
		end
	end
end

== matlab function testEmplanner_cs/Audi_A8_Sedan_1/decision&planning module/EM Planner/calc speed planning start condition ==
  data: plan_start_vx input; plan_start_s_dot output; plan_start_vy input; plan_start_ax input; plan_start_ay input; plan_start_heading input; plan_start_s_dot2 output
function [plan_start_s_dot,plan_start_s_dot2] = fcn(plan_start_vx,plan_start_vy,plan_start_ax,plan_start_ay,plan_start_heading)
% 该函数计算速度规划的初始条件
tor = [cos(plan_start_heading);sin(plan_start_heading)];
v_t = tor'*[plan_start_vx;plan_start_vy];
a_t = tor'*[plan_start_ax;plan_start_ay];
plan_start_s_dot = v_t;
plan_start_s_dot2 = a_t;

== matlab function testEmplanner_cs/Audi_A8_Sedan_1/decision&planning module/EM Planner/genrate index to s ==
  data: path_x input; index2s output; path_y input; origin_x input; origin_y input; origin_match_point_index input
function index2s = fcn(path_x,path_y,origin_x,origin_y,origin_match_point_index)
%该算法将计算法出index和s的转换关系，index2s(i)表示当编号为i时，对应的弧长s
%输入：path_x path_y 待转化的离散点集合
% 	origin_x,origin_y frenet 原点在世界坐标系下的坐标
%   origin_match_point_index 原点的匹配点的编号
% path点的个数
	n = 181;
	index2s = zeros(n,1);
	% 这个循环计算的是以轨迹起点为坐标原点的index2s的转换关系
	for i = 2:181
		index2s(i) = sqrt((path_x(i) - path_x(i-1))^2 + (path_y(i) - path_y(i - 1))^2) + index2s(i-1);
	end
	% 再计算以轨迹起点到frenet_path坐标原点的弧长,记为s0,再用index2s - s0,就得到了以定坐标原点为起点的index2s的关系
	s0 = CalcSFromIndex2S(index2s,path_x,path_y,origin_x,origin_y,origin_match_point_index);
	%计算完s0再用原index2s减去s0
	index2s = index2s - ones(n,1)*s0;
end

function s = CalcSFromIndex2S(index2s,path_x,path_y,proj_x,proj_y,proj_match_point_index)
	%该函数将计算给定的index2s的映射关系后，计算点(proj_x,proj_y)所对应的弧长
	%判断投影点在匹配点的前面还是后面，向量的内积可以判断前后
	vector_1 =[proj_x;proj_y] - [path_x(proj_match_point_index);path_y(proj_match_point_index)];
	if proj_match_point_index < length(path_x)
		vector_2 = [path_x(proj_match_point_index + 1); path_y(proj_match_point_index + 1)] - ...
			[path_x(proj_match_point_index);path_y(proj_match_point_index)];
	else
		vector_2 = [path_x(proj_match_point_index ); path_y(proj_match_point_index )] - ...
			[path_x(proj_match_point_index - 1);path_y(proj_match_point_index - 1)];
	end
	
	if  vector_1' * vector_2 > 0
		%投影点在匹配点的前面
		s = index2s(proj_match_point_index) + sqrt(vector_1'*vector_1);
	else
		%投影点在匹配点的后面
		s = index2s(proj_match_point_index) - sqrt(vector_1'*vector_1);
	end
end

== matlab function testEmplanner_cs/Audi_A8_Sedan_1/decision&planning module/EM Planner/increase st point count ==
  data: s_init input; s output; s_dot_init input; s_dot2_init input; relative_time_init input; s_dot output; s_dot2 output; relative_time output
function [s,s_dot,s_dot2,relative_time] = fcn(s_init,s_dot_init,s_dot2_init,relative_time_init)
%该函数将增密s s_dot s_dot2
% 为什么需要增密，因为控制的执行频率是规划的10倍，轨迹点如果不够密，必然会导致规划效果不好
% 但是若在速度二次规划中点取的太多，会导致二次规划的矩阵规模太大计算太慢
% 所以方法是在二次规划中选取少量的点优化完毕后，在用此函数增密
T = relative_time_init(end);
n = 401;
dt = T/(n-1);
s = zeros(n,1);
s_dot = zeros(n,1);
s_dot2 = zeros(n,1);
relative_time = zeros(n,1);
for i = 1:n
    current_t = (i-1)*dt;
    for j = 1:length(relative_time_init)-1
        if relative_time_init(j) <= current_t && relative_time_init(j+1) > current_t
            break;
        end
    end
    x = current_t - relative_time_init(j);
    s(i) = s_init(j) + s_dot_init(j)*x + (1/3)*s_dot2_init(j)*x^2 + (1/6)*s_dot2_init(j+1)*x^2; 
    s_dot(i) = s_dot_init(j) + 0.5*s_dot2_init(j)*x + 0.5*s_dot2_init(j+1)*x;
    s_dot2(i) = s_dot2_init(j) + (s_dot2_init(j+1) - s_dot2_init(j))*x/(relative_time_init(j+1) - relative_time_init(j));
    relative_time(i) = current_t;
end

== matlab function testEmplanner_cs/Audi_A8_Sedan_1/decision&planning module/EM Planner/obs/Cartesian2Frenet1/Cartesian2Frenet ==
  data: x_set input; s_set output; y_set input; frenet_path_x input; frenet_path_y input; proj_x_set input; proj_y_set input; proj_heading_set input; proj_match_point_index_set input; index2s input; l_set output
function [s_set,l_set] = fcn(x_set,y_set,frenet_path_x,frenet_path_y, ...
	proj_x_set,proj_y_set,proj_heading_set,proj_match_point_index_set,index2s)
	%该函数将计算世界坐标系下的x_set,y_set上的点在frenet_path下的坐标s,l 
	%输入： x_set,y_set 待坐标转换的点
	%       frenet_path_x,frenet_path_y frenet坐标轴
	%       proj_x,proj_y heading ,kappa,proj_match_point_index_set 待坐标转换的点的投影点的信息
	% 		index2s frenet_path 的index与s的转换表

	% 由于不知道有多少个点要做坐标转换，所以需要做缓冲
	n = 128;% 最多处理128个点
	%输出做初始化
	s_set = ones(n,1) * nan;
	l_set = ones(n,1) * nan;
	for i = 1: length(x_set)
		if isnan(x_set(i))
			break;
		end
		
		%计算s,写子函数
		s_set(i) = CalcSFromIndex2S(index2s,frenet_path_x,frenet_path_y,proj_x_set(i),proj_y_set(i),proj_match_point_index_set(i));
		
		%第一章第三节说很详细了，查阅第一章第三节
		n_r = [-sin(proj_heading_set(i));cos(proj_heading_set(i))];
		r_h = [x_set(i);y_set(i)];
		r_r = [proj_x_set(i);proj_y_set(i)];
		l_set(i) = (r_h - r_r)' * n_r;
	end

end


function s = CalcSFromIndex2S(index2s,path_x,path_y,proj_x,proj_y,proj_match_point_index)
	%该函数将计算当指定index2s的映射关系后，计算点proj_x,proj_y的弧长
	vector_1 = [proj_x;proj_y] - [path_x(proj_match_point_index);path_y(proj_match_point_index)];
	%这里要考虑的全面一点，因为要考虑到proj_match_point_index有可能在path的起点或者终点
	if (proj_match_point_index < length(path_x))
		vector_2 = [path_x(proj_match_point_index + 1);path_y(proj_match_point_index + 1)] - ...
			[path_x(proj_match_point_index);path_y(proj_match_point_index)];
	else
		vector_2 = [path_x(proj_match_point_index);path_y(proj_match_point_index)] - ...
			[path_x(proj_match_point_index - 1);path_y(proj_match_point_index - 1)];
	end
	
	if  vector_1' * vector_2 > 0 
		s = index2s(proj_match_point_index) + sqrt(vector_1' * vector_1);
	else
		s = index2s(proj_match_point_index) - sqrt(vector_1' * vector_1);
	end
end

== matlab function testEmplanner_cs/Audi_A8_Sedan_1/decision&planning module/referenceline provider/MATLAB Function1 ==
  data: path_x input; path_heading output; path_y input; path_kappa output
function [path_heading,path_kappa] = fcn(path_x,path_y)
%该函数将计算path的切线方向与x轴的夹角和曲率
%输入：path_x,path_y路径的坐标（全局坐标系下）
%输出：path_heading,path_kappa 路径的heading和曲率
%原理：heading = arctan(dy/dx)
%  kappa = dheading /ds
%  ds = (dx^2 + dy^2)^0.5


%注意，角度的多值性会带来很大的麻烦，需要慎重处理
%例如： x与 x+2*pi代表同一个角度，这种多值性在曲率计算的时候会带来麻烦
%比如： 原本是（0.1 -（-0.1））/ ds,但是如果计算出得-0.1多了一个2*pi
%kappa 就等于(0.1 -(-0.1 + 2*pi)) /ds 曲率就会变得非常大
%还有若采用中点欧拉法计算heading时，即使用 (y2 - y1) / (x2 - x1)的反正切计算一个角度，用(y1 - y0)/(x1 - x0)的反正切
%又计算了一个角度，然后加起来除以2，如果精确值是(a1 + a2)/2,但是最终计算结果可能是(a1 + a2 + 2pi) / 2
%还有tan(x) = tan(x + pi） 所以 arctan(tan(x)) 可能等于x,也可能等于x + pi
%角度的处理非常麻烦，而且角度处理不当往往是许多奇怪错误的源头
%

dx = diff(path_x);
dy = diff(path_y);%计算差分

%用中点欧拉法要比向前欧拉法和向后欧拉法要更精确，但是也可能计算出的结果比精确值多一个pi
%在这里对dx,dy做中点欧拉法，使用四象限反正切计算角度

dx_pre = [dx(1);dx];
dx_after = [dx;dx(end)];
dx_final = (dx_pre + dx_after) / 2;

dy_pre = [dy(1);dy];
dy_after = [dy;dy(end)];
dy_final = (dy_pre + dy_after) / 2;

ds_final = sqrt(dx_final.^2 + dy_final.^2);
path_heading = atan2(dy_final,dx_final);

%atan2(b，a)：4象限反正切，

%　　　　计算b/a对应的反正切值，求点(a，b)对应的角
% 　　　　　(a，b)位于第一象限时，atan2(b，a)取值  0 ~ pi/2
% 　　　　　(a，b)位于第二象限时，atan2(b，a)取值  pi/2 ~ pi
% 　　　　　(a，b)位于第三象限时，atan2(b，a)取值   -pi ~ -pi/2
% 　　　　　(a，b)位于第四象限时，atan2(b，a)取值   -pi/2 ~ 0
%

%中点欧拉法
dheading = diff(path_heading);%差分，size变成length(path_heading) - 1
dheading_pre = [dheading(1);dheading]; %插入一个首元素
dheading_after = [dheading;dheading(end)]; %插入一个尾元素
dheading_final = (dheading_pre + dheading_after) / 2;
%为了防止dheading出现一个2*pi的错误，假设真实的heading较小，用sin(dheading)近似dheading
path_kappa = sin(dheading_final)./ds_final;

== matlab function testEmplanner_cs/Audi_A8_Sedan_1/decision&planning module/EM Planner/obs/Cartesian2Frenet1/MATLAB Function ==
  data: l_set input; s_dot_set output; vx_set input; vy_set input; proj_heading_set input; proj_kappa_set input; l_dot_set output; dl_set output
function [s_dot_set,l_dot_set,dl_set] = fcn(l_set,vx_set,vy_set,proj_heading_set,proj_kappa_set)
%该函数将计算frenet坐标系下的s_dot,l_dot,dl/ds
n = 128;
%输出初始化
s_dot_set = ones(n,1)*nan;
l_dot_set = ones(n,1)*nan;
dl_set = ones(n,1)*nan;

for i = 1: length(l_set)
	if isnan(l_set(i))
		break;
	end
	v_h = [vx_set(i);vy_set(i)];
	n_r = [-sin(proj_heading_set(i));cos(proj_heading_set(i))];
	t_r = [cos(proj_heading_set(i));sin(proj_heading_set(i))];
	l_dot_set(i) = v_h' * n_r;
	s_dot_set(i) = v_h' * t_r /(1-proj_kappa_set(i)*l_set(i));
	%%%% 向量法做cartesian与frenet的转换要简单，但是也有问题，向量法必须依赖速度加速度
	%l' = l_dot / s_dot但是如果s_dot = 0，此方法就失效了
	if abs(s_dot_set(i)) < 1e-6
		dl_set(i) = 0;
	else
		dl_set(i) = l_dot_set(i) / s_dot_set(i);
	end
end

== matlab function testEmplanner_cs/Audi_A8_Sedan_1/decision&planning module/EM Planner/obs/Cartesian2Frenet1/MATLAB Function1 ==
  data: ax_set input; s_dot2_set output; ay_set input; proj_heading_set input; proj_kappa_set input; l_set input; s_dot_set input; dl_set input; l_dot2_set output; ddl_set output
function [s_dot2_set,l_dot2_set,ddl_set] = fcn(ax_set,ay_set,proj_heading_set,proj_kappa_set,l_set,s_dot_set,dl_set)
% 由于不知道有多少个点需要做坐标转换，设一个最大值作为缓冲
 n = 128;
% 输出初始化
s_dot2_set = ones(n,1)*nan;
l_dot2_set = ones(n,1)*nan;
ddl_set = ones(n,1)*nan;

for i = 1 : length(l_set)
	if isnan(l_set(i))
		break;
	end
	a_h = [ax_set(i);ay_set(i)];
	n_r = [-sin(proj_heading_set(i));cos(proj_heading_set(i))];
	t_r = [cos(proj_heading_set(i));sin(proj_heading_set(i))];
	%近似认为 dkr/ds为0 简化计算
	l_dot2_set(i) = a_h' *n_r - proj_kappa_set(i) * (1 - proj_kappa_set(i) * l_set(i)) * s_dot_set(i)^2;
	s_dot2_set(i) = (1/ (1 - proj_kappa_set(i) * l_set(i))) * (a_h' * t_r + 2 * proj_kappa_set(i) * dl_set(i) * s_dot_set(i)^2);
	% 要考虑加速度为0的情况
	if abs(s_dot2_set(i)) < 1e-6
		ddl_set(i) = 0;
	else
		ddl_set(i) = (l_dot2_set(i) - dl_set(i)* s_dot2_set(i)) / (s_dot2_set(i)^2);
	end
end
